simulink model "MSD_model"  (R2021a)
settings: Solver=VariableStepAuto  StartTime=0.0  StopTime=10.0  MaxStep=0.01  RelTol=1e-3
undefined symbols (not defined in the file): b, k, m, x0
settings Model: Creator=46769  LastModifiedBy=46769

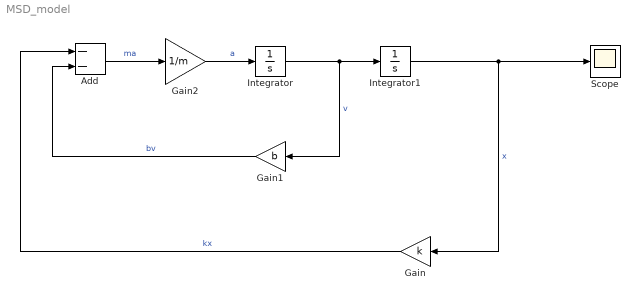
== system MSD_model ==
  Add : Sum  Inputs=--
  Gain : Gain  Gain=k
  Gain1 : Gain  Gain=b
  Gain2 : Gain  Gain=1/m
  Integrator : Integrator
  Integrator1 : Integrator  InitialCondition=x0
  Scope : Scope
  wires:
  Integrator/1 -> Integrator1/1, Gain1/1  "v"
  Integrator1/1 -> Scope/1, Gain/1  "x"
  Gain1/1 -> Add/2  "bv"
  Gain/1 -> Add/1  "kx"
  Gain2/1 -> Integrator/1  "a"
  Add/1 -> Gain2/1  "ma"
